simulink library "DAVS_lib"  (R2022b)
settings: Solver=VariableStepAuto  StartTime=0.0  StopTime=10.0  RelTol=1e-3
undefined symbols (not defined in the file): c0_ne, c0_pe, c_max_ne, c_max_pe, D_ne, D_pe, F, k, N_a_ne, N_a_pe, R_ne, R_pe
libraries: fl_lib x60, nesl_utility x60
(part 1 of 2)
settings Model: Creator=ukeyd  LastModifiedBy=ukeyd

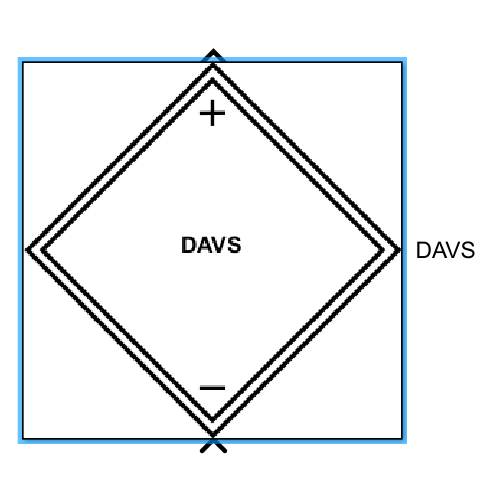
[thumbnail: Simulink's stored preview of the top-level diagram]
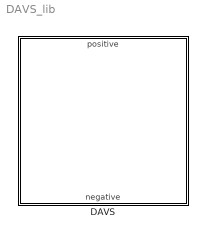
== system DAVS_lib ==
  DAVS : Subsystem  mask{I_app=10}
      mask prompts: I_app "Applied current, I(A):"
      mask init:
      | set_param(gcb,'MaskHideContents','off');
      mask DialogControl DescGroupVar Prompt: Diffusion Aware Voltage Source
      mask DialogControl DescTextVar Prompt: Implements a physics-informed equivalent circuit model that provides a voltage output as a function of lithium concentration in the positive and negative electrodes. It takes the applied current as input in Amperes.
      mask DialogControl ParameterGroupVar Prompt: Input parameters

== system DAVS_lib/DAVS ==
  negative : Inport
  I_app : Subsystem
  OCPne : Subsystem
  OCPpe : Subsystem
  Subtract : Sum  Inputs=+-
  c_surf_ne : Subsystem
  c_surf_pe : Subsystem
  positive : Outport
  wires:
  OCPpe/1(OCP_pe) -> Subtract/1  "OCP_pe"
  Subtract/1 -> positive/1  "OCV"
  OCPne/1(OCP_ne) -> Subtract/2  "OCP_ne"
  I_app/1(Iapp_pe) -> c_surf_pe/1(I_bar(10))
  I_app/2(Iapp_ne) -> c_surf_ne/1(I_bar(10))
  c_surf_pe/1(cse_pe) -> OCPpe/1(cse_pe)
  c_surf_ne/1(cse_ne) -> OCPne/1(cse_ne)

== system DAVS_lib/DAVS/I_app ==
  Clock : Clock
      settings: Decimation=2
  Clock1 : Clock
      settings: Decimation=2
  Constant : Constant  Value=I_app/N_a_pe
  Constant1 : Constant  Value=I_app/N_a_ne
  I_app_ne : MATLAB Function  TreatAsAtomicUnit=on
  I_app_pe : MATLAB Function  TreatAsAtomicUnit=on
  Iapp_pe : Outport
  Iapp_ne : Outport  Port=2
  wires:
  Constant/1 -> I_app_pe/2(I_app)
  Clock/1 -> I_app_pe/1(currentTime)
  I_app_ne/1(signal) -> Iapp_ne/1
  Clock1/1 -> I_app_ne/1(currentTime)
  Constant1/1 -> I_app_ne/2(I_app)
  I_app_pe/1(signal) -> Iapp_pe/1

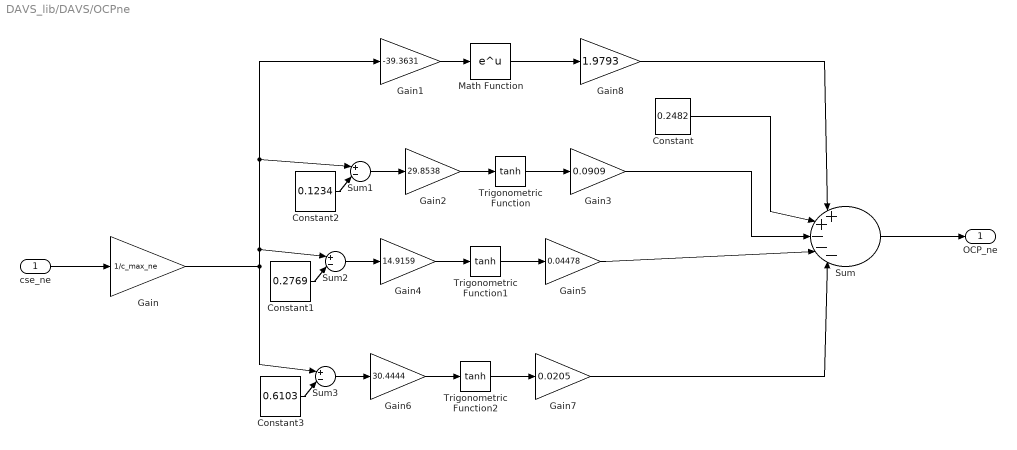
== system DAVS_lib/DAVS/OCPne ==
  cse_ne : Inport
  Constant : Constant  Value=0.2482
  Constant1 : Constant  Value=0.2769
  Constant2 : Constant  Value=0.1234
  Constant3 : Constant  Value=0.6103
  Gain : Gain  Gain=1/c_max_ne
  Gain1 : Gain  Gain=-39.3631
  Gain2 : Gain  Gain=29.8538
  Gain3 : Gain  Gain=0.0909
  Gain4 : Gain  Gain=14.9159
  Gain5 : Gain  Gain=0.04478
  Gain6 : Gain  Gain=30.4444
  Gain7 : Gain  Gain=0.0205
  Gain8 : Gain  Gain=1.9793
  Math Function : Math
  Sum : Sum  Inputs=|++---|
  Sum1 : Sum  Inputs=|+-|
  Sum2 : Sum  Inputs=|+-|
  Sum3 : Sum  Inputs=|+-|
  Trigonometric Function : Trigonometry  Operator=tanh
  Trigonometric Function1 : Trigonometry  Operator=tanh
  Trigonometric Function2 : Trigonometry  Operator=tanh
  OCP_ne : Outport
  wires:
  Gain1/1 -> Math Function/1
  Constant/1 -> Sum/2
  Gain2/1 -> Trigonometric Function/1
  Constant2/1 -> Sum1/2
  Sum1/1 -> Gain2/1
  Trigonometric Function/1 -> Gain3/1
  Gain3/1 -> Sum/3
  Gain5/1 -> Sum/4
  Trigonometric Function1/1 -> Gain5/1
  Sum2/1 -> Gain4/1
  Constant1/1 -> Sum2/2
  Gain4/1 -> Trigonometric Function1/1
  Gain/1 -> Sum1/1, Gain1/1, Sum2/1, Sum3/1
  Gain6/1 -> Trigonometric Function2/1
  Constant3/1 -> Sum3/2
  Sum3/1 -> Gain6/1
  Trigonometric Function2/1 -> Gain7/1
  Gain7/1 -> Sum/5
  Sum/1 -> OCP_ne/1
  Math Function/1 -> Gain8/1
  Gain8/1 -> Sum/1
  cse_ne/1 -> Gain/1

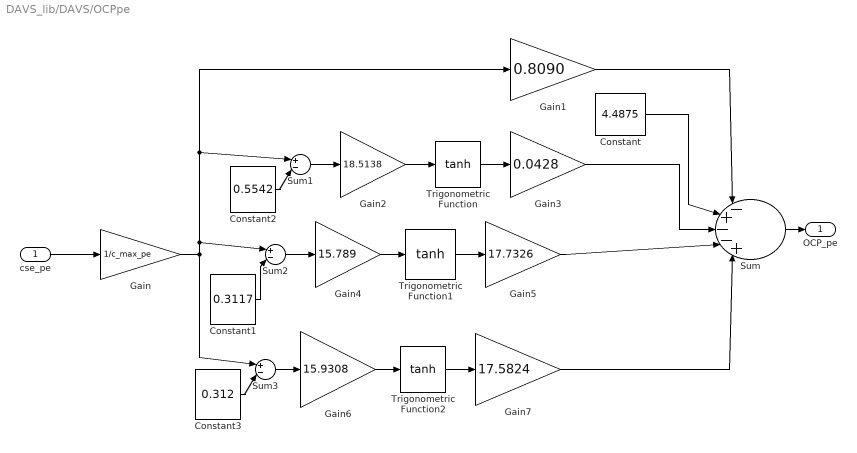
== system DAVS_lib/DAVS/OCPpe ==
  cse_pe : Inport
  Constant : Constant  Value=4.4875
  Constant1 : Constant  Value=0.3117
  Constant2 : Constant  Value=0.5542
  Constant3 : Constant  Value=0.312
  Gain : Gain  Gain=1/c_max_pe
  Gain1 : Gain  Gain=0.8090
  Gain2 : Gain  Gain=18.5138
  Gain3 : Gain  Gain=0.0428
  Gain4 : Gain  Gain=15.789
  Gain5 : Gain  Gain=17.7326
  Gain6 : Gain  Gain=15.9308
  Gain7 : Gain  Gain=17.5824
  Sum : Sum  Inputs=|-+--+|
  Sum1 : Sum  Inputs=|+-|
  Sum2 : Sum  Inputs=|+-|
  Sum3 : Sum  Inputs=|+-|
  Trigonometric Function : Trigonometry  Operator=tanh
  Trigonometric Function1 : Trigonometry  Operator=tanh
  Trigonometric Function2 : Trigonometry  Operator=tanh
  OCP_pe : Outport
  wires:
  Gain1/1 -> Sum/1
  Constant/1 -> Sum/2
  Gain2/1 -> Trigonometric Function/1
  Constant2/1 -> Sum1/2
  Sum1/1 -> Gain2/1
  Trigonometric Function/1 -> Gain3/1
  Gain3/1 -> Sum/3
  Gain5/1 -> Sum/4
  Trigonometric Function1/1 -> Gain5/1
  Sum2/1 -> Gain4/1
  Gain4/1 -> Trigonometric Function1/1
  Gain/1 -> Sum3/1, Sum1/1, Gain1/1, Sum2/1
  Gain6/1 -> Trigonometric Function2/1
  Constant3/1 -> Sum3/2
  Sum3/1 -> Gain6/1
  Trigonometric Function2/1 -> Gain7/1
  Gain7/1 -> Sum/5
  Sum/1 -> OCP_pe/1
  Constant1/1 -> Sum2/2
  cse_pe/1 -> Gain/1

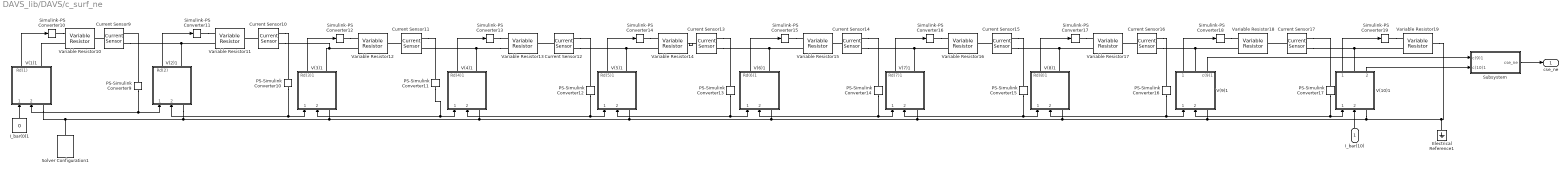
== system DAVS_lib/DAVS/c_surf_ne ==
  I_bar(10) : Inport
  Current Sensor{9..17} (9 alike) : fl_lib/Electrical/Electrical Sensors/Current Sensor
  Electrical Reference1 : fl_lib/Electrical/Electrical Elements/Electrical Reference
  I_bar(0)1 : Constant  Value=0
  PS-Simulink Converter{9..17} (9 alike) : nesl_utility/PS-Simulink Converter  PhysicalDomain=network_engine_domain  SubClassName=ps_output  LeftPortType=input  RightPortType=output  PseudoPeriodic=off  Frequencies=[]  VectorFormat=inherit  Unit=inherit  AffineConversion=off
  Simulink-PS Converter{10..19} (10 alike) : nesl_utility/Simulink-PS Converter  PhysicalDomain=network_engine_domain  SubClassName=ps_input  LeftPortType=input  RightPortType=output  PseudoPeriodic=off  Frequencies=[]  NoiseDistribution=none  NoiseParameters=[]  Unit=1  AffineConversion=off  FilteringAndDerivatives=provide  SimscapeFilterOrder=1  InputFilterTimeConstant=0.001  UdotUserProvided=0
  Solver Configuration1 : nesl_utility/Solver Configuration  PhysicalDomain=network_engine_domain  SubClassName=solver  LeftPortType=input  RightPortType=generic  Tones=[]  Harmonics=[]  SimulateNoise=off  Profile=off  UseLocalSampling=off  EnableSwitchedLinearOptims=on  FrequencyDomain=off  UseCCode=off  RelTol=0.001  AbsTol=0.001  MinStep=1e-09  ToWorkspace=off  RevertToSquareIcSolve=off  NumHomotopyIterations=100  PhasorMode=off  PhasorModeNumHarmonics=1  ConsistencySolver=NEWTON_XTOL_AFTER_FTOL  IndexReductionMethod=DerivativeReplacement  DoDC=off  ResidualTolerance=1e-09  ConsistencyTolSource=GLOBAL  ConsistencyAbsTol=0.001  ConsistencyRelTol=0.001  ConsistencyTolFactor=0.001  UseLocalSolver=off  LocalSolverChoice=NE_BACKWARD_EULER_ADVANCER  ResolveIndetEquations=on  FunctionEvalNumThread=1  LocalSolverSampleTime=0.001  DoFixedCost=off  MaxNonlinIter=3  MaxModeIter=2  ComputeImpulses=off  ImpulseIterations=2  LinearAlgebra=auto  LinearAlgebraNumThread=0  EquationFormulation=NE_TIME_EF  DelaysMemoryBudget=1024  AutomaticFiltering=on  FilteringTimeConstant=0.001  PartitionStorageMethod=AS_NEEDED  PartitionMemoryBudget=1024  PartitionMethod=ROBUST
  Subsystem : Subsystem
  V(1)1 : Subsystem
  V(10)1 : Subsystem
      settings: PortSchema="{\"entries\":[{\"content\":{\"sides\":[{\"content\":{\"connectorIds\":[\"In1\",\"In2\",\"LConn1\"]},\"type\":\"ConnectorPlacement.EquallySpacedRectSide\",\"uuid\":\"326f821b-4aa4-48b5-a56d-533981abc63c\"},{\"content\":{\"connectorIds\":[\"Out1\",\"RConn1\",\"Out2\"],\"side\":\"RIGHT\"},\"type\":\"ConnectorPlacement.EquallySpacedRectSide\",\"uuid\":\"b0236978-0a5d-48ca-88e9-ee638761e80f\"},{\"content\":{\"connectorIds\":[],\"side\":\"TOP\"},\"type\":\"ConnectorPlacement.EquallySpacedRectSide\",\"uuid\":\"04a39df3-4241-4fd8-817b-894698047bcb\"}]},\"type\":\"ConnectorPlacement.EquallySpacedConnector\",\"uuid\":\"2275d19c-d06f-40ec-b16a-f4e76404e636\"}],\"packageUris\":[\"http://schema.mathworks.com/mf0/Connector/R2020b\"],\"version\":\"1.0\"}"
  V(2)1 : Subsystem
  V(3)1 : Subsystem
  V(4)1 : Subsystem
  V(5)1 : Subsystem
  V(6)1 : Subsystem
  V(7)1 : Subsystem
  V(8)1 : Subsystem
  V(9)1 : Subsystem
      settings: PortSchema="{\"entries\":[{\"content\":{\"sides\":[{\"content\":{\"connectorIds\":[\"In1\",\"In2\",\"LConn1\"]},\"type\":\"ConnectorPlacement.EquallySpacedRectSide\",\"uuid\":\"326f821b-4aa4-48b5-a56d-533981abc63c\"},{\"content\":{\"connectorIds\":[\"Out1\",\"RConn1\",\"Out2\"],\"side\":\"RIGHT\"},\"type\":\"ConnectorPlacement.EquallySpacedRectSide\",\"uuid\":\"b0236978-0a5d-48ca-88e9-ee638761e80f\"},{\"content\":{\"connectorIds\":[],\"side\":\"TOP\"},\"type\":\"ConnectorPlacement.EquallySpacedRectSide\",\"uuid\":\"04a39df3-4241-4fd8-817b-894698047bcb\"}]},\"type\":\"ConnectorPlacement.EquallySpacedConnector\",\"uuid\":\"2275d19c-d06f-40ec-b16a-f4e76404e636\"}],\"packageUris\":[\"http://schema.mathworks.com/mf0/Connector/R2020b\"],\"version\":\"1.0\"}"
  Variable Resistor{10..19} (10 alike) : fl_lib/Electrical/Electrical Elements/Variable Resistor  Rmin=0 Ohm  i_specify=off  i_priority=None  i=0 A  i_nominal_specify=off  i_nominal_unit=A  i_nominal_value=1  v_specify=off  v_priority=None  v=0 V  v_nominal_specify=off  v_nominal_unit=V  v_nominal_value=1
  cse_ne : Outport
  wires:
  PS-Simulink Converter16/1 -> V(9)1/1(I_bar(8)), V(8)1/2(I_bar(8))
  I_bar(0)1/1 -> V(1)1/1(I_bar(0))
  V(7)1/1(Rd(7)1) -> Simulink-PS Converter16/1
  V(2)1/1(Rd(2)) -> Simulink-PS Converter11/1
  PS-Simulink Converter15/1 -> V(8)1/1(I_bar(7)), V(7)1/2(I_bar(7))
  V(8)1/1(Rd(8)1) -> Simulink-PS Converter17/1
  PS-Simulink Converter11/1 -> V(3)1/2(I_bar(3)), V(4)1/1(I_bar(3))
  V(4)1/1(Rd(4)1) -> Simulink-PS Converter13/1
  PS-Simulink Converter12/1 -> V(5)1/1(I_bar(4)), V(4)1/2(I_bar(4))
  PS-Simulink Converter10/1 -> V(3)1/1(I_bar(2)), V(2)1/2(I_bar(2))
  V(9)1/1(Rd(9)1) -> Simulink-PS Converter18/1
  V(3)1/1(Rd(3)1) -> Simulink-PS Converter12/1
  V(1)1/1(Rd(1)) -> Simulink-PS Converter10/1
  PS-Simulink Converter13/1 -> V(6)1/1(I_bar(5)), V(5)1/2(I_bar(5))
  V(5)1/1(Rd(5)1) -> Simulink-PS Converter14/1
  V(6)1/1(Rd(6)1) -> Simulink-PS Converter15/1
  I_bar(10)/1 -> V(10)1/2(I_bar(10))
  PS-Simulink Converter14/1 -> V(7)1/1(I_bar(6)), V(6)1/2(I_bar(6))
  PS-Simulink Converter17/1 -> V(10)1/1(I_bar(9)), V(9)1/2(I_bar(9))
  PS-Simulink Converter9/1 -> V(1)1/2(I_bar(1)), V(2)1/1(I_bar(1))
  V(10)1/1(Rd(9)1) -> Simulink-PS Converter19/1
  V(10)1/2(c(10)1) -> Subsystem/2(c(10)1)
  V(9)1/2(c(9)1) -> Subsystem/1(c(9)1)
  Subsystem/1(cse_ne) -> cse_ne/1
  connections:
  Solver Configuration1/RConn1 -- V(2)1/LConn1 -- V(3)1/LConn1 -- V(4)1/LConn1 -- Electrical Reference1/LConn1 -- Variable Resistor19/RConn1 -- V(10)1/LConn1 -- V(9)1/LConn1 -- V(8)1/LConn1 -- V(7)1/LConn1 -- V(6)1/LConn1 -- V(5)1/LConn1 -- V(1)1/LConn1
  Simulink-PS Converter11/RConn1 -- Variable Resistor11/LConn1
  Variable Resistor17/LConn2 -- V(8)1/RConn1 -- Current Sensor15/RConn2
  Current Sensor13/LConn1 -- Variable Resistor14/RConn1
  Current Sensor16/RConn2 -- V(9)1/RConn1 -- Variable Resistor18/LConn2
  Variable Resistor14/LConn2 -- V(5)1/RConn1 -- Current Sensor12/RConn2
  Simulink-PS Converter13/RConn1 -- Variable Resistor13/LConn1
  Current Sensor10/RConn1 -- PS-Simulink Converter10/LConn1
  Simulink-PS Converter12/RConn1 -- Variable Resistor12/LConn1
  PS-Simulink Converter9/LConn1 -- Current Sensor9/RConn1
  Current Sensor12/RConn1 -- PS-Simulink Converter12/LConn1
  Variable Resistor16/LConn2 -- V(7)1/RConn1 -- Current Sensor14/RConn2
  Current Sensor11/LConn1 -- Variable Resistor12/RConn1
  Current Sensor17/RConn1 -- PS-Simulink Converter17/LConn1
  Variable Resistor15/LConn2 -- V(6)1/RConn1 -- Current Sensor13/RConn2
  Current Sensor10/LConn1 -- Variable Resistor11/RConn1
  Current Sensor11/RConn1 -- PS-Simulink Converter11/LConn1
  Current Sensor15/RConn1 -- PS-Simulink Converter15/LConn1
  Current Sensor14/RConn1 -- PS-Simulink Converter14/LConn1
  Current Sensor17/RConn2 -- Variable Resistor19/LConn2 -- V(10)1/RConn1
  Current Sensor10/RConn2 -- Variable Resistor12/LConn2 -- V(3)1/RConn1
  Simulink-PS Converter10/RConn1 -- Variable Resistor10/LConn1
  Current Sensor16/RConn1 -- PS-Simulink Converter16/LConn1
  Variable Resistor11/LConn2 -- V(2)1/RConn1 -- Current Sensor9/RConn2
  Current Sensor15/LConn1 -- Variable Resistor16/RConn1
  Variable Resistor13/LConn2 -- Current Sensor11/RConn2 -- V(4)1/RConn1
  Simulink-PS Converter14/RConn1 -- Variable Resistor14/LConn1
  V(1)1/RConn1 -- Variable Resistor10/LConn2
  Current Sensor12/LConn1 -- Variable Resistor13/RConn1
  Current Sensor14/LConn1 -- Variable Resistor15/RConn1
  Simulink-PS Converter19/RConn1 -- Variable Resistor19/LConn1
  Current Sensor17/LConn1 -- Variable Resistor18/RConn1
  Current Sensor16/LConn1 -- Variable Resistor17/RConn1
  Current Sensor9/LConn1 -- Variable Resistor10/RConn1
  Simulink-PS Converter15/RConn1 -- Variable Resistor15/LConn1
  Simulink-PS Converter17/RConn1 -- Variable Resistor17/LConn1
  Simulink-PS Converter18/RConn1 -- Variable Resistor18/LConn1
  Simulink-PS Converter16/RConn1 -- Variable Resistor16/LConn1
  Current Sensor13/RConn1 -- PS-Simulink Converter13/LConn1

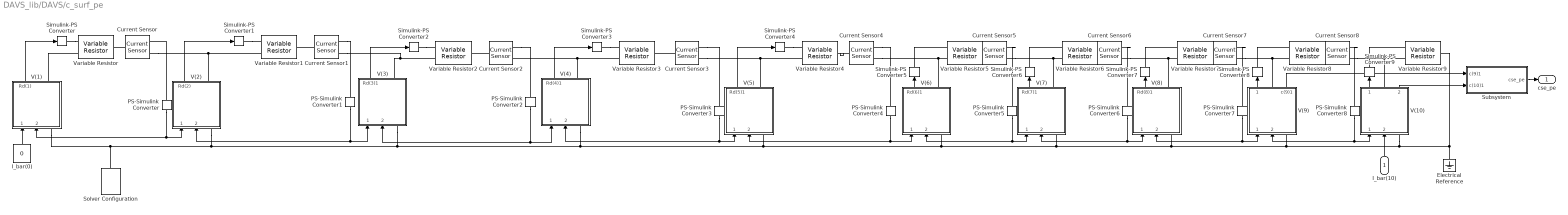
== system DAVS_lib/DAVS/c_surf_pe ==
  I_bar(10) : Inport
  Current Sensor{,1..8} (9 alike) : fl_lib/Electrical/Electrical Sensors/Current Sensor
  Electrical Reference : fl_lib/Electrical/Electrical Elements/Electrical Reference
  I_bar(0) : Constant  Value=0
  PS-Simulink Converter{,1..8} (9 alike) : nesl_utility/PS-Simulink Converter  PhysicalDomain=network_engine_domain  SubClassName=ps_output  LeftPortType=input  RightPortType=output  PseudoPeriodic=off  Frequencies=[]  VectorFormat=inherit  Unit=inherit  AffineConversion=off
  Simulink-PS Converter{,1..9} (10 alike) : nesl_utility/Simulink-PS Converter  PhysicalDomain=network_engine_domain  SubClassName=ps_input  LeftPortType=input  RightPortType=output  PseudoPeriodic=off  Frequencies=[]  NoiseDistribution=none  NoiseParameters=[]  Unit=1  AffineConversion=off  FilteringAndDerivatives=provide  SimscapeFilterOrder=1  InputFilterTimeConstant=0.001  UdotUserProvided=0
  Solver Configuration : nesl_utility/Solver Configuration  PhysicalDomain=network_engine_domain  SubClassName=solver  LeftPortType=input  RightPortType=generic  Tones=[]  Harmonics=[]  SimulateNoise=off  Profile=off  UseLocalSampling=off  EnableSwitchedLinearOptims=on  FrequencyDomain=off  UseCCode=off  RelTol=0.001  AbsTol=0.001  MinStep=1e-09  ToWorkspace=off  RevertToSquareIcSolve=off  NumHomotopyIterations=100  PhasorMode=off  PhasorModeNumHarmonics=1  ConsistencySolver=NEWTON_XTOL_AFTER_FTOL  IndexReductionMethod=DerivativeReplacement  DoDC=off  ResidualTolerance=1e-09  ConsistencyTolSource=GLOBAL  ConsistencyAbsTol=0.001  ConsistencyRelTol=0.001  ConsistencyTolFactor=0.001  UseLocalSolver=off  LocalSolverChoice=NE_BACKWARD_EULER_ADVANCER  ResolveIndetEquations=on  FunctionEvalNumThread=1  LocalSolverSampleTime=0.001  DoFixedCost=off  MaxNonlinIter=3  MaxModeIter=2  ComputeImpulses=off  ImpulseIterations=2  LinearAlgebra=auto  LinearAlgebraNumThread=0  EquationFormulation=NE_TIME_EF  DelaysMemoryBudget=1024  AutomaticFiltering=on  FilteringTimeConstant=0.001  PartitionStorageMethod=AS_NEEDED  PartitionMemoryBudget=1024  PartitionMethod=ROBUST
  Subsystem : Subsystem
  V(1) : Subsystem
  V(10) : Subsystem
      settings: PortSchema="{\"entries\":[{\"content\":{\"sides\":[{\"content\":{\"connectorIds\":[\"In1\",\"In2\",\"LConn1\"]},\"type\":\"ConnectorPlacement.EquallySpacedRectSide\",\"uuid\":\"326f821b-4aa4-48b5-a56d-533981abc63c\"},{\"content\":{\"connectorIds\":[\"Out1\",\"RConn1\",\"Out2\"],\"side\":\"RIGHT\"},\"type\":\"ConnectorPlacement.EquallySpacedRectSide\",\"uuid\":\"b0236978-0a5d-48ca-88e9-ee638761e80f\"},{\"content\":{\"connectorIds\":[],\"side\":\"TOP\"},\"type\":\"ConnectorPlacement.EquallySpacedRectSide\",\"uuid\":\"04a39df3-4241-4fd8-817b-894698047bcb\"}]},\"type\":\"ConnectorPlacement.EquallySpacedConnector\",\"uuid\":\"2275d19c-d06f-40ec-b16a-f4e76404e636\"}],\"packageUris\":[\"http://schema.mathworks.com/mf0/Connector/R2020b\"],\"version\":\"1.0\"}"
  V(2) : Subsystem
  V(3) : Subsystem
  V(4) : Subsystem
  V(5) : Subsystem
  V(6) : Subsystem
  V(7) : Subsystem
  V(8) : Subsystem
  V(9) : Subsystem
      settings: PortSchema="{\"entries\":[{\"content\":{\"sides\":[{\"content\":{\"connectorIds\":[\"In1\",\"In2\",\"LConn1\"]},\"type\":\"ConnectorPlacement.EquallySpacedRectSide\",\"uuid\":\"326f821b-4aa4-48b5-a56d-533981abc63c\"},{\"content\":{\"connectorIds\":[\"Out1\",\"RConn1\",\"Out2\"],\"side\":\"RIGHT\"},\"type\":\"ConnectorPlacement.EquallySpacedRectSide\",\"uuid\":\"b0236978-0a5d-48ca-88e9-ee638761e80f\"},{\"content\":{\"connectorIds\":[],\"side\":\"TOP\"},\"type\":\"ConnectorPlacement.EquallySpacedRectSide\",\"uuid\":\"04a39df3-4241-4fd8-817b-894698047bcb\"}]},\"type\":\"ConnectorPlacement.EquallySpacedConnector\",\"uuid\":\"2275d19c-d06f-40ec-b16a-f4e76404e636\"}],\"packageUris\":[\"http://schema.mathworks.com/mf0/Connector/R2020b\"],\"version\":\"1.0\"}"
  Variable Resistor{,1..9} (10 alike) : fl_lib/Electrical/Electrical Elements/Variable Resistor  Rmin=0 Ohm  i_specify=off  i_priority=None  i=0 A  i_nominal_specify=off  i_nominal_unit=A  i_nominal_value=1  v_specify=off  v_priority=None  v=0 V  v_nominal_specify=off  v_nominal_unit=V  v_nominal_value=1
  cse_pe : Outport
  wires:
  PS-Simulink Converter5/1 -> V(6)/2(I_bar(6)), V(7)/1(I_bar(6))
  V(4)/1(Rd(4)1) -> Simulink-PS Converter3/1
  PS-Simulink Converter2/1 -> V(4)/1(I_bar(3)), V(3)/2(I_bar(3))
  V(2)/1(Rd(2)) -> Simulink-PS Converter1/1
  V(5)/1(Rd(5)1) -> Simulink-PS Converter4/1
  PS-Simulink Converter6/1 -> V(7)/2(I_bar(7)), V(8)/1(I_bar(7))
  PS-Simulink Converter1/1 -> V(2)/2(I_bar(2)), V(3)/1(I_bar(2))
  PS-Simulink Converter3/1 -> V(4)/2(I_bar(4)), V(5)/1(I_bar(4))
  PS-Simulink Converter7/1 -> V(8)/2(I_bar(8)), V(9)/1(I_bar(8))
  I_bar(0)/1 -> V(1)/1(I_bar(0))
  V(1)/1(Rd(1)) -> Simulink-PS Converter/1
  PS-Simulink Converter4/1 -> V(5)/2(I_bar(5)), V(6)/1(I_bar(5))
  PS-Simulink Converter8/1 -> V(9)/2(I_bar(9)), V(10)/1(I_bar(9))
  V(3)/1(Rd(3)1) -> Simulink-PS Converter2/1
  PS-Simulink Converter/1 -> V(2)/1(I_bar(1)), V(1)/2(I_bar(1))
  I_bar(10)/1 -> V(10)/2(I_bar(10))
  V(6)/1(Rd(6)1) -> Simulink-PS Converter5/1
  V(7)/1(Rd(7)1) -> Simulink-PS Converter6/1
  V(8)/1(Rd(8)1) -> Simulink-PS Converter7/1
  V(9)/1(Rd(9)1) -> Simulink-PS Converter8/1
  V(10)/1(Rd(9)1) -> Simulink-PS Converter9/1
  V(9)/2(c(9)1) -> Subsystem/1(c(9)1)
  Subsystem/1(cse_pe) -> cse_pe/1
  V(10)/2(c(10)1) -> Subsystem/2(c(10)1)
  connections:
  Variable Resistor6/LConn2 -- Current Sensor5/RConn2 -- V(7)/RConn1
  Simulink-PS Converter6/RConn1 -- Variable Resistor6/LConn1
  Simulink-PS Converter/RConn1 -- Variable Resistor/LConn1
  Variable Resistor4/LConn2 -- Current Sensor3/RConn2 -- V(5)/RConn1
  Simulink-PS Converter4/RConn1 -- Variable Resistor4/LConn1
  Current Sensor5/LConn1 -- Variable Resistor5/RConn1
  Simulink-PS Converter5/RConn1 -- Variable Resistor5/LConn1
  Variable Resistor7/LConn2 -- Current Sensor6/RConn2 -- V(8)/RConn1
  Variable Resistor5/LConn2 -- Current Sensor4/RConn2 -- V(6)/RConn1
  Current Sensor1/LConn1 -- Variable Resistor1/RConn1
  Simulink-PS Converter3/RConn1 -- Variable Resistor3/LConn1
  Current Sensor2/LConn1 -- Variable Resistor2/RConn1
  Simulink-PS Converter1/RConn1 -- Variable Resistor1/LConn1
  V(5)/LConn1 -- Electrical Reference/LConn1 -- Variable Resistor9/RConn1 -- V(10)/LConn1 -- V(9)/LConn1 -- V(8)/LConn1 -- V(7)/LConn1 -- V(6)/LConn1 -- V(4)/LConn1 -- V(3)/LConn1 -- V(2)/LConn1 -- V(1)/LConn1 -- Solver Configuration/RConn1
  Current Sensor/LConn1 -- Variable Resistor/RConn1
  PS-Simulink Converter/LConn1 -- Current Sensor/RConn1
  Current Sensor4/RConn1 -- PS-Simulink Converter4/LConn1
  V(4)/RConn1 -- Variable Resistor3/LConn2 -- Current Sensor2/RConn2
  Current Sensor6/LConn1 -- Variable Resistor6/RConn1
  Variable Resistor9/LConn2 -- V(10)/RConn1 -- Current Sensor8/RConn2
  Current Sensor3/RConn1 -- PS-Simulink Converter3/LConn1
  Current Sensor3/LConn1 -- Variable Resistor3/RConn1
  Current Sensor1/RConn1 -- PS-Simulink Converter1/LConn1
  Current Sensor4/LConn1 -- Variable Resistor4/RConn1
  Variable Resistor1/LConn2 -- Current Sensor/RConn2 -- V(2)/RConn1
  Simulink-PS Converter8/RConn1 -- Variable Resistor8/LConn1
  V(1)/RConn1 -- Variable Resistor/LConn2
  Variable Resistor2/LConn2 -- Current Sensor1/RConn2 -- V(3)/RConn1
  Simulink-PS Converter9/RConn1 -- Variable Resistor9/LConn1
  Variable Resistor8/LConn2 -- Current Sensor7/RConn2 -- V(9)/RConn1
  Simulink-PS Converter2/RConn1 -- Variable Resistor2/LConn1
  Current Sensor7/LConn1 -- Variable Resistor7/RConn1
  Current Sensor2/RConn1 -- PS-Simulink Converter2/LConn1
  Current Sensor8/LConn1 -- Variable Resistor8/RConn1
  Current Sensor5/RConn1 -- PS-Simulink Converter5/LConn1
  Current Sensor6/RConn1 -- PS-Simulink Converter6/LConn1
  Variable Resistor7/LConn1 -- Simulink-PS Converter7/RConn1
  Current Sensor7/RConn1 -- PS-Simulink Converter7/LConn1
  Current Sensor8/RConn1 -- PS-Simulink Converter8/LConn1

== system DAVS_lib/DAVS/c_surf_ne/Subsystem ==
  c(9)1 : Inport
  c(10)1 : Inport  Port=2
  Gain : Gain  Gain=0.5
  Gain1 : Gain  Gain=1.5
  Sum : Sum  Inputs=|+-|
  cse_ne : Outport
  wires:
  c(9)1/1 -> Gain/1
  c(10)1/1 -> Gain1/1
  Gain/1 -> Sum/2
  Gain1/1 -> Sum/1
  Sum/1 -> cse_ne/1

== system DAVS_lib/DAVS/c_surf_ne/V(1)1 ==
  I_bar(0) : Inport
  I_bar(1) : Inport  Port=2
  Controlled Voltage Source : fl_lib/Electrical/Electrical Sources/Controlled Voltage Source
  I(1) : Subsystem
  Simulink-PS Converter : nesl_utility/Simulink-PS Converter  PhysicalDomain=network_engine_domain  SubClassName=ps_input  LeftPortType=input  RightPortType=output  PseudoPeriodic=off  Frequencies=[]  NoiseDistribution=none  NoiseParameters=[]  Unit=1  AffineConversion=off  FilteringAndDerivatives=provide  SimscapeFilterOrder=1  InputFilterTimeConstant=0.001  UdotUserProvided=0
  Subsystem1 : Subsystem
  V(1) : Subsystem
  c(1) : Subsystem
  n : Constant
  + : PMIOPort  Tag=PMCPort  Side=Right
  - : PMIOPort  Tag=PMCPort  Port=2  Side=Left
  Rd(1) : Outport
  wires:
  Subsystem1/1(Rd) -> Rd(1)/1
  n/1 -> c(1)/2(n), Subsystem1/1(n)
  I_bar(0)/1 -> I(1)/1(I_bar(0))
  V(1)/1(V(1)) -> Simulink-PS Converter/1
  c(1)/1(c(1)) -> V(1)/1(c(1))
  I_bar(1)/1 -> I(1)/2(I_bar(1))
  I(1)/1(I(1)) -> c(1)/1(I(1))
  connections:
  -/RConn1 -- Controlled Voltage Source/RConn2
  +/RConn1 -- Controlled Voltage Source/LConn1
  Simulink-PS Converter/RConn1 -- Controlled Voltage Source/RConn1

== system DAVS_lib/DAVS/c_surf_ne/V(10)1 ==
  I_bar(9) : Inport
  I_bar(10) : Inport  Port=2
  Controlled Voltage Source : fl_lib/Electrical/Electrical Sources/Controlled Voltage Source
  I(10) : Subsystem
  Simulink-PS Converter : nesl_utility/Simulink-PS Converter  PhysicalDomain=network_engine_domain  SubClassName=ps_input  LeftPortType=input  RightPortType=output  PseudoPeriodic=off  Frequencies=[]  NoiseDistribution=none  NoiseParameters=[]  Unit=1  AffineConversion=off  FilteringAndDerivatives=provide  SimscapeFilterOrder=1  InputFilterTimeConstant=0.001  UdotUserProvided=0
  Subsystem1 : Subsystem
  V(10) : Subsystem
  c(10) : Subsystem
  n : Constant  Value=10
  - : PMIOPort  Tag=PMCPort  Side=Left
  + : PMIOPort  Tag=PMCPort  Port=2  Side=Right
  Rd(9)1 : Outport
  c(10)1 : Outport  Port=2
  wires:
  n/1 -> Subsystem1/1(n), c(10)/2(n)
  Subsystem1/1(Rd) -> Rd(9)1/1
  V(10)/1(V(10)) -> Simulink-PS Converter/1
  I(10)/1(I(10)) -> c(10)/1(I(10))
  I_bar(10)/1 -> I(10)/2(I_bar(10))
  c(10)/1(c(10)) -> V(10)/1(c(10)), c(10)1/1
  I_bar(9)/1 -> I(10)/1(I_bar(9))
  connections:
  Simulink-PS Converter/RConn1 -- Controlled Voltage Source/RConn1
  -/RConn1 -- Controlled Voltage Source/RConn2
  +/RConn1 -- Controlled Voltage Source/LConn1

== system DAVS_lib/DAVS/c_surf_ne/V(2)1 ==
  I_bar(1) : Inport
  I_bar(2) : Inport  Port=2
  Controlled Voltage Source : fl_lib/Electrical/Electrical Sources/Controlled Voltage Source
  I(2) : Subsystem
  Simulink-PS Converter : nesl_utility/Simulink-PS Converter  PhysicalDomain=network_engine_domain  SubClassName=ps_input  LeftPortType=input  RightPortType=output  PseudoPeriodic=off  Frequencies=[]  NoiseDistribution=none  NoiseParameters=[]  Unit=1  AffineConversion=off  FilteringAndDerivatives=provide  SimscapeFilterOrder=1  InputFilterTimeConstant=0.001  UdotUserProvided=0
  Subsystem1 : Subsystem
  V(2) : Subsystem
  c(2) : Subsystem
  n : Constant  Value=2
  + : PMIOPort  Tag=PMCPort  Side=Right
  - : PMIOPort  Tag=PMCPort  Port=2  Side=Left
  Rd(2) : Outport
  wires:
  n/1 -> Subsystem1/1(n), c(2)/2(n)
  Subsystem1/1(Rd) -> Rd(2)/1
  V(2)/1(V(2)) -> Simulink-PS Converter/1
  I(2)/1(I(2)) -> c(2)/1(I(2))
  I_bar(2)/1 -> I(2)/2(I_bar(2))
  c(2)/1(c(2)) -> V(2)/1(c(2))
  I_bar(1)/1 -> I(2)/1(I_bar(1))
  connections:
  -/RConn1 -- Controlled Voltage Source/RConn2
  Simulink-PS Converter/RConn1 -- Controlled Voltage Source/RConn1
  +/RConn1 -- Controlled Voltage Source/LConn1

== system DAVS_lib/DAVS/c_surf_ne/V(3)1 ==
  I_bar(2) : Inport
  I_bar(3) : Inport  Port=2
  Controlled Voltage Source : fl_lib/Electrical/Electrical Sources/Controlled Voltage Source
  I(3) : Subsystem
  Simulink-PS Converter : nesl_utility/Simulink-PS Converter  PhysicalDomain=network_engine_domain  SubClassName=ps_input  LeftPortType=input  RightPortType=output  PseudoPeriodic=off  Frequencies=[]  NoiseDistribution=none  NoiseParameters=[]  Unit=1  AffineConversion=off  FilteringAndDerivatives=provide  SimscapeFilterOrder=1  InputFilterTimeConstant=0.001  UdotUserProvided=0
  Subsystem1 : Subsystem
  V(3) : Subsystem
  c(3) : Subsystem
  n : Constant  Value=3
  + : PMIOPort  Tag=PMCPort  Side=Right
  - : PMIOPort  Tag=PMCPort  Port=2  Side=Left
  Rd(3)1 : Outport
  wires:
  n/1 -> Subsystem1/1(n), c(3)/2(n)
  Subsystem1/1(Rd) -> Rd(3)1/1
  V(3)/1(V(3)) -> Simulink-PS Converter/1
  I_bar(2)/1 -> I(3)/1(I_bar(2))
  c(3)/1(c(3)) -> V(3)/1(c(3))
  I_bar(3)/1 -> I(3)/2(I_bar(3))
  I(3)/1(I(3)) -> c(3)/1(I(3))
  connections:
  Simulink-PS Converter/RConn1 -- Controlled Voltage Source/RConn1
  -/RConn1 -- Controlled Voltage Source/RConn2
  +/RConn1 -- Controlled Voltage Source/LConn1

== system DAVS_lib/DAVS/c_surf_ne/V(4)1 ==
  I_bar(3) : Inport
  I_bar(4) : Inport  Port=2
  Controlled Voltage Source : fl_lib/Electrical/Electrical Sources/Controlled Voltage Source
  I(4) : Subsystem
  Simulink-PS Converter : nesl_utility/Simulink-PS Converter  PhysicalDomain=network_engine_domain  SubClassName=ps_input  LeftPortType=input  RightPortType=output  PseudoPeriodic=off  Frequencies=[]  NoiseDistribution=none  NoiseParameters=[]  Unit=1  AffineConversion=off  FilteringAndDerivatives=provide  SimscapeFilterOrder=1  InputFilterTimeConstant=0.001  UdotUserProvided=0
  Subsystem1 : Subsystem
  V(4) : Subsystem
  c(4) : Subsystem
  n : Constant  Value=4
  + : PMIOPort  Tag=PMCPort  Side=Right
  - : PMIOPort  Tag=PMCPort  Port=2  Side=Left
  Rd(4)1 : Outport
  wires:
  Subsystem1/1(Rd) -> Rd(4)1/1
  n/1 -> Subsystem1/1(n), c(4)/2(n)
  V(4)/1(V(4)) -> Simulink-PS Converter/1
  I(4)/1(I(4)) -> c(4)/1(I(4))
  I_bar(4)/1 -> I(4)/2(I_bar(4))
  c(4)/1(c(4)) -> V(4)/1(c(4))
  I_bar(3)/1 -> I(4)/1(I_bar(3))
  connections:
  +/RConn1 -- Controlled Voltage Source/LConn1
  Simulink-PS Converter/RConn1 -- Controlled Voltage Source/RConn1
  -/RConn1 -- Controlled Voltage Source/RConn2

== system DAVS_lib/DAVS/c_surf_ne/V(5)1 ==
  I_bar(4) : Inport
  I_bar(5) : Inport  Port=2
  Controlled Voltage Source : fl_lib/Electrical/Electrical Sources/Controlled Voltage Source
  I(n) : Subsystem
  Simulink-PS Converter : nesl_utility/Simulink-PS Converter  PhysicalDomain=network_engine_domain  SubClassName=ps_input  LeftPortType=input  RightPortType=output  PseudoPeriodic=off  Frequencies=[]  NoiseDistribution=none  NoiseParameters=[]  Unit=1  AffineConversion=off  FilteringAndDerivatives=provide  SimscapeFilterOrder=1  InputFilterTimeConstant=0.001  UdotUserProvided=0
  Subsystem1 : Subsystem
  V(5) : Subsystem
  c(5) : Subsystem
  n : Constant  Value=5
  + : PMIOPort  Tag=PMCPort  Side=Right
  - : PMIOPort  Tag=PMCPort  Port=2  Side=Left
  Rd(5)1 : Outport
  wires:
  n/1 -> Subsystem1/1(n), c(5)/2(n)
  Subsystem1/1(Rd) -> Rd(5)1/1
  V(5)/1(V(5)) -> Simulink-PS Converter/1
  I_bar(4)/1 -> I(n)/1(I_bar(4))
  c(5)/1(c(5)) -> V(5)/1(c(5))
  I_bar(5)/1 -> I(n)/2(I_bar(5))
  I(n)/1(I(5)) -> c(5)/1(I(5))
  connections:
  -/RConn1 -- Controlled Voltage Source/RConn2
  +/RConn1 -- Controlled Voltage Source/LConn1
  Simulink-PS Converter/RConn1 -- Controlled Voltage Source/RConn1

== system DAVS_lib/DAVS/c_surf_ne/V(6)1 ==
  I_bar(5) : Inport
  I_bar(6) : Inport  Port=2
  Controlled Voltage Source : fl_lib/Electrical/Electrical Sources/Controlled Voltage Source
  I(6) : Subsystem
  Simulink-PS Converter : nesl_utility/Simulink-PS Converter  PhysicalDomain=network_engine_domain  SubClassName=ps_input  LeftPortType=input  RightPortType=output  PseudoPeriodic=off  Frequencies=[]  NoiseDistribution=none  NoiseParameters=[]  Unit=1  AffineConversion=off  FilteringAndDerivatives=provide  SimscapeFilterOrder=1  InputFilterTimeConstant=0.001  UdotUserProvided=0
  Subsystem1 : Subsystem
  V(6) : Subsystem
  c(6) : Subsystem
  n : Constant  Value=6
  + : PMIOPort  Tag=PMCPort  Side=Right
  - : PMIOPort  Tag=PMCPort  Port=2  Side=Left
  Rd(6)1 : Outport
  wires:
  Subsystem1/1(Rd) -> Rd(6)1/1
  n/1 -> Subsystem1/1(n), c(6)/2(n)
  V(6)/1(V(6)) -> Simulink-PS Converter/1
  I(6)/1(I(6)) -> c(6)/1(I(6))
  I_bar(6)/1 -> I(6)/2(I_bar(5))
  c(6)/1(c(6)) -> V(6)/1(c(6))
  I_bar(5)/1 -> I(6)/1(I_bar(6))
  connections:
  Simulink-PS Converter/RConn1 -- Controlled Voltage Source/RConn1
  -/RConn1 -- Controlled Voltage Source/RConn2
  +/RConn1 -- Controlled Voltage Source/LConn1

== system DAVS_lib/DAVS/c_surf_ne/V(7)1 ==
  I_bar(6) : Inport
  I_bar(7) : Inport  Port=2
  Controlled Voltage Source : fl_lib/Electrical/Electrical Sources/Controlled Voltage Source
  I(7) : Subsystem
  Simulink-PS Converter : nesl_utility/Simulink-PS Converter  PhysicalDomain=network_engine_domain  SubClassName=ps_input  LeftPortType=input  RightPortType=output  PseudoPeriodic=off  Frequencies=[]  NoiseDistribution=none  NoiseParameters=[]  Unit=1  AffineConversion=off  FilteringAndDerivatives=provide  SimscapeFilterOrder=1  InputFilterTimeConstant=0.001  UdotUserProvided=0
  Subsystem1 : Subsystem
  V(7) : Subsystem
  c(7) : Subsystem
  n : Constant  Value=7
  + : PMIOPort  Tag=PMCPort  Side=Right
  - : PMIOPort  Tag=PMCPort  Port=2  Side=Left
  Rd(7)1 : Outport
  wires:
  Subsystem1/1(Rd) -> Rd(7)1/1
  n/1 -> Subsystem1/1(n), c(7)/2(n)
  V(7)/1(V(7)) -> Simulink-PS Converter/1
  I_bar(6)/1 -> I(7)/1(I_bar(6))
  c(7)/1(c(7)) -> V(7)/1(c(7))
  I_bar(7)/1 -> I(7)/2(I_bar(7))
  I(7)/1(I(7)) -> c(7)/1(I(7))
  connections:
  -/RConn1 -- Controlled Voltage Source/RConn2
  +/RConn1 -- Controlled Voltage Source/LConn1
  Simulink-PS Converter/RConn1 -- Controlled Voltage Source/RConn1

== system DAVS_lib/DAVS/c_surf_ne/V(8)1 ==
  I_bar(7) : Inport
  I_bar(8) : Inport  Port=2
  Controlled Voltage Source : fl_lib/Electrical/Electrical Sources/Controlled Voltage Source
  I(8) : Subsystem
  Simulink-PS Converter : nesl_utility/Simulink-PS Converter  PhysicalDomain=network_engine_domain  SubClassName=ps_input  LeftPortType=input  RightPortType=output  PseudoPeriodic=off  Frequencies=[]  NoiseDistribution=none  NoiseParameters=[]  Unit=1  AffineConversion=off  FilteringAndDerivatives=provide  SimscapeFilterOrder=1  InputFilterTimeConstant=0.001  UdotUserProvided=0
  Subsystem1 : Subsystem
  V(8) : Subsystem
  c(1) : Subsystem
  n : Constant  Value=8
  + : PMIOPort  Tag=PMCPort  Side=Right
  - : PMIOPort  Tag=PMCPort  Port=2  Side=Left
  Rd(8)1 : Outport
  wires:
  n/1 -> Subsystem1/1(n), c(1)/2(n)
  Subsystem1/1(Rd) -> Rd(8)1/1
  V(8)/1(V(8)) -> Simulink-PS Converter/1
  I(8)/1(I(8)) -> c(1)/1(I(8))
  I_bar(8)/1 -> I(8)/2(I_bar(8))
  c(1)/1(c(8)) -> V(8)/1(c(8))
  I_bar(7)/1 -> I(8)/1(I_bar(7))
  connections:
  Simulink-PS Converter/RConn1 -- Controlled Voltage Source/RConn1
  +/RConn1 -- Controlled Voltage Source/LConn1
  -/RConn1 -- Controlled Voltage Source/RConn2

== system DAVS_lib/DAVS/c_surf_ne/V(9)1 ==
  I_bar(8) : Inport
  I_bar(9) : Inport  Port=2
  Controlled Voltage Source : fl_lib/Electrical/Electrical Sources/Controlled Voltage Source
  I(9) : Subsystem
  Simulink-PS Converter : nesl_utility/Simulink-PS Converter  PhysicalDomain=network_engine_domain  SubClassName=ps_input  LeftPortType=input  RightPortType=output  PseudoPeriodic=off  Frequencies=[]  NoiseDistribution=none  NoiseParameters=[]  Unit=1  AffineConversion=off  FilteringAndDerivatives=provide  SimscapeFilterOrder=1  InputFilterTimeConstant=0.001  UdotUserProvided=0
  Subsystem1 : Subsystem
  V(9) : Subsystem
  c(9) : Subsystem
  n : Constant  Value=9
  - : PMIOPort  Tag=PMCPort  Side=Left
  + : PMIOPort  Tag=PMCPort  Port=2  Side=Right
  Rd(9)1 : Outport
  c(9)1 : Outport  Port=2
  wires:
  Subsystem1/1(Rd) -> Rd(9)1/1
  n/1 -> Subsystem1/1(n), c(9)/2(n)
  V(9)/1(V(9)) -> Simulink-PS Converter/1
  I_bar(8)/1 -> I(9)/1(I_bar(8))
  c(9)/1(c(9)) -> V(9)/1(c(9)), c(9)1/1
  I_bar(9)/1 -> I(9)/2(I_bar(9))
  I(9)/1(I(9)) -> c(9)/1(I(9))
  connections:
  +/RConn1 -- Controlled Voltage Source/LConn1
  -/RConn1 -- Controlled Voltage Source/RConn2
  Simulink-PS Converter/RConn1 -- Controlled Voltage Source/RConn1

== system DAVS_lib/DAVS/c_surf_pe/Subsystem ==
  c(9)1 : Inport
  c(10)1 : Inport  Port=2
  Gain : Gain  Gain=0.5
  Gain1 : Gain  Gain=1.5
  Sum : Sum  Inputs=|+-|
  cse_pe : Outport
  wires:
  c(9)1/1 -> Gain/1
  c(10)1/1 -> Gain1/1
  Gain/1 -> Sum/2
  Gain1/1 -> Sum/1
  Sum/1 -> cse_pe/1

== system DAVS_lib/DAVS/c_surf_pe/V(1) ==
  I_bar(0) : Inport
  I_bar(1) : Inport  Port=2
  Controlled Voltage Source : fl_lib/Electrical/Electrical Sources/Controlled Voltage Source
  I(1) : Subsystem
  Simulink-PS Converter : nesl_utility/Simulink-PS Converter  PhysicalDomain=network_engine_domain  SubClassName=ps_input  LeftPortType=input  RightPortType=output  PseudoPeriodic=off  Frequencies=[]  NoiseDistribution=none  NoiseParameters=[]  Unit=1  AffineConversion=off  FilteringAndDerivatives=provide  SimscapeFilterOrder=1  InputFilterTimeConstant=0.001  UdotUserProvided=0
  Subsystem1 : Subsystem
  V(1) : Subsystem
  c(1) : Subsystem
  n : Constant
  + : PMIOPort  Tag=PMCPort  Side=Right
  - : PMIOPort  Tag=PMCPort  Port=2  Side=Left
  Rd(1) : Outport
  wires:
  I(1)/1(I(1)) -> c(1)/1(I(1))
  I_bar(1)/1 -> I(1)/2(I_bar(1))
  c(1)/1(c(1)) -> V(1)/1(c(1))
  V(1)/1(V(1)) -> Simulink-PS Converter/1
  I_bar(0)/1 -> I(1)/1(I_bar(0))
  n/1 -> Subsystem1/1(n), c(1)/2(n)
  Subsystem1/1(Rd) -> Rd(1)/1
  connections:
  Simulink-PS Converter/RConn1 -- Controlled Voltage Source/RConn1
  +/RConn1 -- Controlled Voltage Source/LConn1
  -/RConn1 -- Controlled Voltage Source/RConn2

== system DAVS_lib/DAVS/c_surf_pe/V(10) ==
  I_bar(9) : Inport
  I_bar(10) : Inport  Port=2
  Controlled Voltage Source : fl_lib/Electrical/Electrical Sources/Controlled Voltage Source
  I(10) : Subsystem
  Simulink-PS Converter : nesl_utility/Simulink-PS Converter  PhysicalDomain=network_engine_domain  SubClassName=ps_input  LeftPortType=input  RightPortType=output  PseudoPeriodic=off  Frequencies=[]  NoiseDistribution=none  NoiseParameters=[]  Unit=1  AffineConversion=off  FilteringAndDerivatives=provide  SimscapeFilterOrder=1  InputFilterTimeConstant=0.001  UdotUserProvided=0
  Subsystem1 : Subsystem
  V(10) : Subsystem
  c(10) : Subsystem
  n : Constant  Value=10
  - : PMIOPort  Tag=PMCPort  Side=Left
  + : PMIOPort  Tag=PMCPort  Port=2  Side=Right
  Rd(9)1 : Outport
  c(10)1 : Outport  Port=2
  wires:
  I_bar(9)/1 -> I(10)/1(I_bar(9))
  c(10)/1(c(10)) -> c(10)1/1, V(10)/1(c(10))
  I_bar(10)/1 -> I(10)/2(I_bar(10))
  I(10)/1(I(10)) -> c(10)/1(I(10))
  V(10)/1(V(10)) -> Simulink-PS Converter/1
  Subsystem1/1(Rd) -> Rd(9)1/1
  n/1 -> c(10)/2(n), Subsystem1/1(n)
  connections:
  +/RConn1 -- Controlled Voltage Source/LConn1
  -/RConn1 -- Controlled Voltage Source/RConn2
  Simulink-PS Converter/RConn1 -- Controlled Voltage Source/RConn1

== system DAVS_lib/DAVS/c_surf_pe/V(2) ==
  I_bar(1) : Inport
  I_bar(2) : Inport  Port=2
  Controlled Voltage Source : fl_lib/Electrical/Electrical Sources/Controlled Voltage Source
  I(2) : Subsystem
  Simulink-PS Converter : nesl_utility/Simulink-PS Converter  PhysicalDomain=network_engine_domain  SubClassName=ps_input  LeftPortType=input  RightPortType=output  PseudoPeriodic=off  Frequencies=[]  NoiseDistribution=none  NoiseParameters=[]  Unit=1  AffineConversion=off  FilteringAndDerivatives=provide  SimscapeFilterOrder=1  InputFilterTimeConstant=0.001  UdotUserProvided=0
  Subsystem1 : Subsystem
  V(2) : Subsystem
  c(2) : Subsystem
  n : Constant  Value=2
  + : PMIOPort  Tag=PMCPort  Side=Right
  - : PMIOPort  Tag=PMCPort  Port=2  Side=Left
  Rd(2) : Outport
  wires:
  I_bar(1)/1 -> I(2)/1(I_bar(1))
  c(2)/1(c(2)) -> V(2)/1(c(2))
  I_bar(2)/1 -> I(2)/2(I_bar(2))
  I(2)/1(I(2)) -> c(2)/1(I(2))
  V(2)/1(V(2)) -> Simulink-PS Converter/1
  Subsystem1/1(Rd) -> Rd(2)/1
  n/1 -> c(2)/2(n), Subsystem1/1(n)
  connections:
  +/RConn1 -- Controlled Voltage Source/LConn1
  Simulink-PS Converter/RConn1 -- Controlled Voltage Source/RConn1
  -/RConn1 -- Controlled Voltage Source/RConn2

== system DAVS_lib/DAVS/c_surf_pe/V(3) ==
  I_bar(2) : Inport
  I_bar(3) : Inport  Port=2
  Controlled Voltage Source : fl_lib/Electrical/Electrical Sources/Controlled Voltage Source
  I(3) : Subsystem
  Simulink-PS Converter : nesl_utility/Simulink-PS Converter  PhysicalDomain=network_engine_domain  SubClassName=ps_input  LeftPortType=input  RightPortType=output  PseudoPeriodic=off  Frequencies=[]  NoiseDistribution=none  NoiseParameters=[]  Unit=1  AffineConversion=off  FilteringAndDerivatives=provide  SimscapeFilterOrder=1  InputFilterTimeConstant=0.001  UdotUserProvided=0
  Subsystem1 : Subsystem
  V(3) : Subsystem
  c(3) : Subsystem
  n : Constant  Value=3
  + : PMIOPort  Tag=PMCPort  Side=Right
  - : PMIOPort  Tag=PMCPort  Port=2  Side=Left
  Rd(3)1 : Outport
  wires:
  I(3)/1(I(3)) -> c(3)/1(I(3))
  I_bar(3)/1 -> I(3)/2(I_bar(3))
  c(3)/1(c(3)) -> V(3)/1(c(3))
  I_bar(2)/1 -> I(3)/1(I_bar(2))
  V(3)/1(V(3)) -> Simulink-PS Converter/1
  Subsystem1/1(Rd) -> Rd(3)1/1
  n/1 -> c(3)/2(n), Subsystem1/1(n)
  connections:
  +/RConn1 -- Controlled Voltage Source/LConn1
  -/RConn1 -- Controlled Voltage Source/RConn2
  Simulink-PS Converter/RConn1 -- Controlled Voltage Source/RConn1

== system DAVS_lib/DAVS/c_surf_pe/V(4) ==
  I_bar(3) : Inport
  I_bar(4) : Inport  Port=2
  Controlled Voltage Source : fl_lib/Electrical/Electrical Sources/Controlled Voltage Source
  I(4) : Subsystem
  Simulink-PS Converter : nesl_utility/Simulink-PS Converter  PhysicalDomain=network_engine_domain  SubClassName=ps_input  LeftPortType=input  RightPortType=output  PseudoPeriodic=off  Frequencies=[]  NoiseDistribution=none  NoiseParameters=[]  Unit=1  AffineConversion=off  FilteringAndDerivatives=provide  SimscapeFilterOrder=1  InputFilterTimeConstant=0.001  UdotUserProvided=0
  Subsystem1 : Subsystem
  V(4) : Subsystem
  c(4) : Subsystem
  n : Constant  Value=4
  + : PMIOPort  Tag=PMCPort  Side=Right
  - : PMIOPort  Tag=PMCPort  Port=2  Side=Left
  Rd(4)1 : Outport
  wires:
  I_bar(3)/1 -> I(4)/1(I_bar(3))
  c(4)/1(c(4)) -> V(4)/1(c(4))
  I_bar(4)/1 -> I(4)/2(I_bar(4))
  I(4)/1(I(4)) -> c(4)/1(I(4))
  V(4)/1(V(4)) -> Simulink-PS Converter/1
  n/1 -> c(4)/2(n), Subsystem1/1(n)
  Subsystem1/1(Rd) -> Rd(4)1/1
  connections:
  -/RConn1 -- Controlled Voltage Source/RConn2
  Simulink-PS Converter/RConn1 -- Controlled Voltage Source/RConn1
  +/RConn1 -- Controlled Voltage Source/LConn1

== system DAVS_lib/DAVS/c_surf_pe/V(5) ==
  I_bar(4) : Inport
  I_bar(5) : Inport  Port=2
  Controlled Voltage Source : fl_lib/Electrical/Electrical Sources/Controlled Voltage Source
  I(n) : Subsystem
  Simulink-PS Converter : nesl_utility/Simulink-PS Converter  PhysicalDomain=network_engine_domain  SubClassName=ps_input  LeftPortType=input  RightPortType=output  PseudoPeriodic=off  Frequencies=[]  NoiseDistribution=none  NoiseParameters=[]  Unit=1  AffineConversion=off  FilteringAndDerivatives=provide  SimscapeFilterOrder=1  InputFilterTimeConstant=0.001  UdotUserProvided=0
  Subsystem1 : Subsystem
  V(5) : Subsystem
  c(5) : Subsystem
  n : Constant  Value=5
  + : PMIOPort  Tag=PMCPort  Side=Right
  - : PMIOPort  Tag=PMCPort  Port=2  Side=Left
  Rd(5)1 : Outport
  wires:
  I(n)/1(I(5)) -> c(5)/1(I(5))
  I_bar(5)/1 -> I(n)/2(I_bar(5))
  c(5)/1(c(5)) -> V(5)/1(c(5))
  I_bar(4)/1 -> I(n)/1(I_bar(4))
  V(5)/1(V(5)) -> Simulink-PS Converter/1
  Subsystem1/1(Rd) -> Rd(5)1/1
  n/1 -> c(5)/2(n), Subsystem1/1(n)
  connections:
  Simulink-PS Converter/RConn1 -- Controlled Voltage Source/RConn1
  +/RConn1 -- Controlled Voltage Source/LConn1
  -/RConn1 -- Controlled Voltage Source/RConn2

== system DAVS_lib/DAVS/c_surf_pe/V(6) ==
  I_bar(5) : Inport
  I_bar(6) : Inport  Port=2
  Controlled Voltage Source : fl_lib/Electrical/Electrical Sources/Controlled Voltage Source
  I(6) : Subsystem
  Simulink-PS Converter : nesl_utility/Simulink-PS Converter  PhysicalDomain=network_engine_domain  SubClassName=ps_input  LeftPortType=input  RightPortType=output  PseudoPeriodic=off  Frequencies=[]  NoiseDistribution=none  NoiseParameters=[]  Unit=1  AffineConversion=off  FilteringAndDerivatives=provide  SimscapeFilterOrder=1  InputFilterTimeConstant=0.001  UdotUserProvided=0
  Subsystem1 : Subsystem
  V(6) : Subsystem
  c(6) : Subsystem
  n : Constant  Value=6
  + : PMIOPort  Tag=PMCPort  Side=Right
  - : PMIOPort  Tag=PMCPort  Port=2  Side=Left
  Rd(6)1 : Outport
  wires:
  I_bar(5)/1 -> I(6)/1(I_bar(6))
  c(6)/1(c(6)) -> V(6)/1(c(6))
  I_bar(6)/1 -> I(6)/2(I_bar(5))
  I(6)/1(I(6)) -> c(6)/1(I(6))
  V(6)/1(V(6)) -> Simulink-PS Converter/1
  n/1 -> c(6)/2(n), Subsystem1/1(n)
  Subsystem1/1(Rd) -> Rd(6)1/1
  connections:
  +/RConn1 -- Controlled Voltage Source/LConn1
  -/RConn1 -- Controlled Voltage Source/RConn2
  Simulink-PS Converter/RConn1 -- Controlled Voltage Source/RConn1

== system DAVS_lib/DAVS/c_surf_pe/V(7) ==
  I_bar(6) : Inport
  I_bar(7) : Inport  Port=2
  Controlled Voltage Source : fl_lib/Electrical/Electrical Sources/Controlled Voltage Source
  I(7) : Subsystem
  Simulink-PS Converter : nesl_utility/Simulink-PS Converter  PhysicalDomain=network_engine_domain  SubClassName=ps_input  LeftPortType=input  RightPortType=output  PseudoPeriodic=off  Frequencies=[]  NoiseDistribution=none  NoiseParameters=[]  Unit=1  AffineConversion=off  FilteringAndDerivatives=provide  SimscapeFilterOrder=1  InputFilterTimeConstant=0.001  UdotUserProvided=0
  Subsystem1 : Subsystem
  V(7) : Subsystem
  c(7) : Subsystem
  n : Constant  Value=7
  + : PMIOPort  Tag=PMCPort  Side=Right
  - : PMIOPort  Tag=PMCPort  Port=2  Side=Left
  Rd(7)1 : Outport
  wires:
  I(7)/1(I(7)) -> c(7)/1(I(7))
  I_bar(7)/1 -> I(7)/2(I_bar(7))
  c(7)/1(c(7)) -> V(7)/1(c(7))
  I_bar(6)/1 -> I(7)/1(I_bar(6))
  V(7)/1(V(7)) -> Simulink-PS Converter/1
  n/1 -> c(7)/2(n), Subsystem1/1(n)
  Subsystem1/1(Rd) -> Rd(7)1/1
  connections:
  Simulink-PS Converter/RConn1 -- Controlled Voltage Source/RConn1
  +/RConn1 -- Controlled Voltage Source/LConn1
  -/RConn1 -- Controlled Voltage Source/RConn2

== system DAVS_lib/DAVS/c_surf_pe/V(8) ==
  I_bar(7) : Inport
  I_bar(8) : Inport  Port=2
  Controlled Voltage Source : fl_lib/Electrical/Electrical Sources/Controlled Voltage Source
  I(8) : Subsystem
  Simulink-PS Converter : nesl_utility/Simulink-PS Converter  PhysicalDomain=network_engine_domain  SubClassName=ps_input  LeftPortType=input  RightPortType=output  PseudoPeriodic=off  Frequencies=[]  NoiseDistribution=none  NoiseParameters=[]  Unit=1  AffineConversion=off  FilteringAndDerivatives=provide  SimscapeFilterOrder=1  InputFilterTimeConstant=0.001  UdotUserProvided=0
  Subsystem1 : Subsystem
  V(8) : Subsystem
  c(1) : Subsystem
  n : Constant  Value=8
  + : PMIOPort  Tag=PMCPort  Side=Right
  - : PMIOPort  Tag=PMCPort  Port=2  Side=Left
  Rd(8)1 : Outport
  wires:
  I_bar(7)/1 -> I(8)/1(I_bar(7))
  c(1)/1(c(8)) -> V(8)/1(c(8))
  I_bar(8)/1 -> I(8)/2(I_bar(8))
  I(8)/1(I(8)) -> c(1)/1(I(8))
  V(8)/1(V(8)) -> Simulink-PS Converter/1
  Subsystem1/1(Rd) -> Rd(8)1/1
  n/1 -> c(1)/2(n), Subsystem1/1(n)
  connections:
  -/RConn1 -- Controlled Voltage Source/RConn2
  +/RConn1 -- Controlled Voltage Source/LConn1
  Simulink-PS Converter/RConn1 -- Controlled Voltage Source/RConn1

== system DAVS_lib/DAVS/c_surf_pe/V(9) ==
  I_bar(8) : Inport
  I_bar(9) : Inport  Port=2
  Controlled Voltage Source : fl_lib/Electrical/Electrical Sources/Controlled Voltage Source
  I(9) : Subsystem
  Simulink-PS Converter : nesl_utility/Simulink-PS Converter  PhysicalDomain=network_engine_domain  SubClassName=ps_input  LeftPortType=input  RightPortType=output  PseudoPeriodic=off  Frequencies=[]  NoiseDistribution=none  NoiseParameters=[]  Unit=1  AffineConversion=off  FilteringAndDerivatives=provide  SimscapeFilterOrder=1  InputFilterTimeConstant=0.001  UdotUserProvided=0
  Subsystem1 : Subsystem
  V(9) : Subsystem
  c(9) : Subsystem
  n : Constant  Value=9
  - : PMIOPort  Tag=PMCPort  Side=Left
  + : PMIOPort  Tag=PMCPort  Port=2  Side=Right
  Rd(9)1 : Outport
  c(9)1 : Outport  Port=2
  wires:
  I(9)/1(I(9)) -> c(9)/1(I(9))
  I_bar(9)/1 -> I(9)/2(I_bar(9))
  c(9)/1(c(9)) -> c(9)1/1, V(9)/1(c(9))
  I_bar(8)/1 -> I(9)/1(I_bar(8))
  V(9)/1(V(9)) -> Simulink-PS Converter/1
  n/1 -> c(9)/2(n), Subsystem1/1(n)
  Subsystem1/1(Rd) -> Rd(9)1/1
  connections:
  Simulink-PS Converter/RConn1 -- Controlled Voltage Source/RConn1
  -/RConn1 -- Controlled Voltage Source/RConn2
  +/RConn1 -- Controlled Voltage Source/LConn1

== system DAVS_lib/DAVS/c_surf_ne/V(1)1/I(1) ==
  I_bar(0) : Inport
  I_bar(1) : Inport  Port=2
  Sum : Sum  Inputs=|-+|
  I(1) : Outport
  wires:
  Sum/1 -> I(1)/1
  I_bar(0)/1 -> Sum/2
  I_bar(1)/1 -> Sum/1

== system DAVS_lib/DAVS/c_surf_ne/V(1)1/Subsystem1 ==
  n : Inport
  Constant : Constant  Value=2
  Constant1 : Constant  Value=10
  Divide : Product  Inputs=*/
  Gain : Gain  Gain=k
  Gain1 : Gain  Gain=4*pi*R_ne*D_ne
  Math Function : Math  Operator=pow
  Rd : Outport
  wires:
  Constant1/1 -> Gain/1
  Divide/1 -> Rd/1
  Math Function/1 -> Gain1/1
  Gain1/1 -> Divide/2
  Constant/1 -> Math Function/2
  Gain/1 -> Divide/1
  n/1 -> Math Function/1

== system DAVS_lib/DAVS/c_surf_ne/V(1)1/V(1) ==
  c(1) : Inport
  Gain : Gain  Gain=k*F
  V(1) : Outport
  wires:
  Gain/1 -> V(1)/1
  c(1)/1 -> Gain/1

== system DAVS_lib/DAVS/c_surf_ne/V(1)1/c(1) ==
  I(1) : Inport
  n : Inport  Port=2
  Divide : Product  Inputs=*/
  Gain : Gain  Gain=F
  Integrator : Integrator  InitialCondition=c0_ne
  Subsystem : Subsystem
  c(1) : Outport
  wires:
  n/1 -> Subsystem/1(n)
  Subsystem/1(dV(n)) -> Gain/1
  Integrator/1 -> c(1)/1
  Divide/1 -> Integrator/1
  Gain/1 -> Divide/2
  I(1)/1 -> Divide/1

== system DAVS_lib/DAVS/c_surf_ne/V(10)1/I(10) ==
  I_bar(9) : Inport
  I_bar(10) : Inport  Port=2
  Sum : Sum  Inputs=|-+|
  I(10) : Outport
  wires:
  I_bar(10)/1 -> Sum/1
  I_bar(9)/1 -> Sum/2
  Sum/1 -> I(10)/1

== system DAVS_lib/DAVS/c_surf_ne/V(10)1/Subsystem1 ==
  n : Inport
  Constant : Constant  Value=2
  Constant1 : Constant  Value=10
  Divide : Product  Inputs=*/
  Gain : Gain  Gain=k
  Gain1 : Gain  Gain=4*pi*R_ne*D_ne
  Math Function : Math  Operator=pow
  Rd : Outport
  wires:
  Constant1/1 -> Gain/1
  Divide/1 -> Rd/1
  Math Function/1 -> Gain1/1
  Gain1/1 -> Divide/2
  Constant/1 -> Math Function/2
  Gain/1 -> Divide/1
  n/1 -> Math Function/1

== system DAVS_lib/DAVS/c_surf_ne/V(10)1/V(10) ==
  c(10) : Inport
  Gain : Gain  Gain=k*F
  V(10) : Outport
  wires:
  c(10)/1 -> Gain/1
  Gain/1 -> V(10)/1

== system DAVS_lib/DAVS/c_surf_ne/V(10)1/c(10) ==
  I(10) : Inport
  n : Inport  Port=2
  Divide : Product  Inputs=*/
  Gain : Gain  Gain=F
  Integrator : Integrator  InitialCondition=c0_ne
  Subsystem : Subsystem
  c(10) : Outport
  wires:
  Subsystem/1(dV(n)1) -> Gain/1
  n/1 -> Subsystem/1(n1)
  I(10)/1 -> Divide/1
  Gain/1 -> Divide/2
  Divide/1 -> Integrator/1
  Integrator/1 -> c(10)/1

== system DAVS_lib/DAVS/c_surf_ne/V(2)1/I(2) ==
  I_bar(1) : Inport
  I_bar(2) : Inport  Port=2
  Sum : Sum  Inputs=|-+|
  I(2) : Outport
  wires:
  I_bar(2)/1 -> Sum/1
  I_bar(1)/1 -> Sum/2
  Sum/1 -> I(2)/1

== system DAVS_lib/DAVS/c_surf_ne/V(2)1/Subsystem1 ==
  n : Inport
  Constant : Constant  Value=2
  Constant1 : Constant  Value=10
  Divide : Product  Inputs=*/
  Gain : Gain  Gain=k
  Gain1 : Gain  Gain=4*pi*R_ne*D_ne
  Math Function : Math  Operator=pow
  Rd : Outport
  wires:
  Constant1/1 -> Gain/1
  Divide/1 -> Rd/1
  Math Function/1 -> Gain1/1
  Gain1/1 -> Divide/2
  Constant/1 -> Math Function/2
  Gain/1 -> Divide/1
  n/1 -> Math Function/1

== system DAVS_lib/DAVS/c_surf_ne/V(2)1/V(2) ==
  c(2) : Inport
  Gain : Gain  Gain=k*F
  V(2) : Outport
  wires:
  c(2)/1 -> Gain/1
  Gain/1 -> V(2)/1

== system DAVS_lib/DAVS/c_surf_ne/V(2)1/c(2) ==
  I(2) : Inport
  n : Inport  Port=2
  Divide : Product  Inputs=*/
  Gain : Gain  Gain=F
  Integrator : Integrator  InitialCondition=c0_ne
  Subsystem : Subsystem
  c(2) : Outport
  wires:
  Subsystem/1(dV(n)1) -> Gain/1
  n/1 -> Subsystem/1(n1)
  I(2)/1 -> Divide/1
  Gain/1 -> Divide/2
  Divide/1 -> Integrator/1
  Integrator/1 -> c(2)/1

== system DAVS_lib/DAVS/c_surf_ne/V(3)1/I(3) ==
  I_bar(2) : Inport
  I_bar(3) : Inport  Port=2
  Sum : Sum  Inputs=|-+|
  I(3) : Outport
  wires:
  Sum/1 -> I(3)/1
  I_bar(2)/1 -> Sum/2
  I_bar(3)/1 -> Sum/1

== system DAVS_lib/DAVS/c_surf_ne/V(3)1/Subsystem1 ==
  n : Inport
  Constant : Constant  Value=2
  Constant1 : Constant  Value=10
  Divide : Product  Inputs=*/
  Gain : Gain  Gain=k
  Gain1 : Gain  Gain=4*pi*R_ne*D_ne
  Math Function : Math  Operator=pow
  Rd : Outport
  wires:
  Constant1/1 -> Gain/1
  Divide/1 -> Rd/1
  Math Function/1 -> Gain1/1
  Gain1/1 -> Divide/2
  Constant/1 -> Math Function/2
  Gain/1 -> Divide/1
  n/1 -> Math Function/1

== system DAVS_lib/DAVS/c_surf_ne/V(3)1/V(3) ==
  c(3) : Inport
  Gain : Gain  Gain=k*F
  V(3) : Outport
  wires:
  Gain/1 -> V(3)/1
  c(3)/1 -> Gain/1
